simulink model "te_plant_network_controller"  (R2013b)
settings: Solver=ode5  SolverMode=SingleTasking  StartTime=0.0  StopTime=inf  FixedStep=Ts_base  MaxStep=Ts_base  MinStep=1e-6  RelTol=1e-6
InitFcn:
  | global model_type
  | model_type = 0
  | 
  | init_model
StopFcn:
  | %TEplot
values from neighbouring files (symbols this model uses):
  Dprocplc = 0    [init_model.m]
  Ts_actuator = repmat(Ts_scan,12,1)    [init_model.m]
  Ts_save = Ts_base    (= 0.000277777777778)    [init_model.m]
  Ts_scan = 30*Ts_base    (= 0.00833333333333)    [init_model.m]
  Ts_sensor = repmat(Ts_scan,41,1)    [init_model.m]
  xmeas_local_port_rx = xmeas_local_port_tx    [init_model.m]
  xmeas_local_port_tx = 9601:9699    [init_model.m]
  xmv_local_port_rx = xmv_local_port_tx    [init_model.m]
  xmv_local_port_tx = 9801:9899    [init_model.m]
libraries: TEsim_utils x8
settings Model: Creator=rnc4  LastModifiedBy=rnc4
settings DataIOCC: LimitDataPoints=off  LoadInitialState=on  SaveFinalState=on  SaveFormat=Structure  SignalLoggingSaveFormat=ModelDataLogs  SaveOutput=off  SaveTime=off  SignalLoggingName=sigsOut
settings OptimizationCC: InitFltsAndDblsToZero=on  SimCompilerOptimization=On
settings DebuggingCC: SaveWithParameterizedLinksMsg=none  SignalResolutionControl=TryResolveAllWithWarning  SolverPrmCheckMsg=none  MultiTaskDSMMsg=warning  MultiTaskCondExecSysMsg=none  FcnCallInpInsideContextMsg=UseLocalSettings
settings HardwareCC: TargetUnknown=on
settings RTWCC: IncludeERTFirstTime=on
settings GRTTargetCC: TargetFcnLib=ansi_tfl_tmw.mat  CodeReplacementLibrary=None  CombineOutputUpdateFcns=off  CPPClassGenCompliant=on  GRTInterface=on

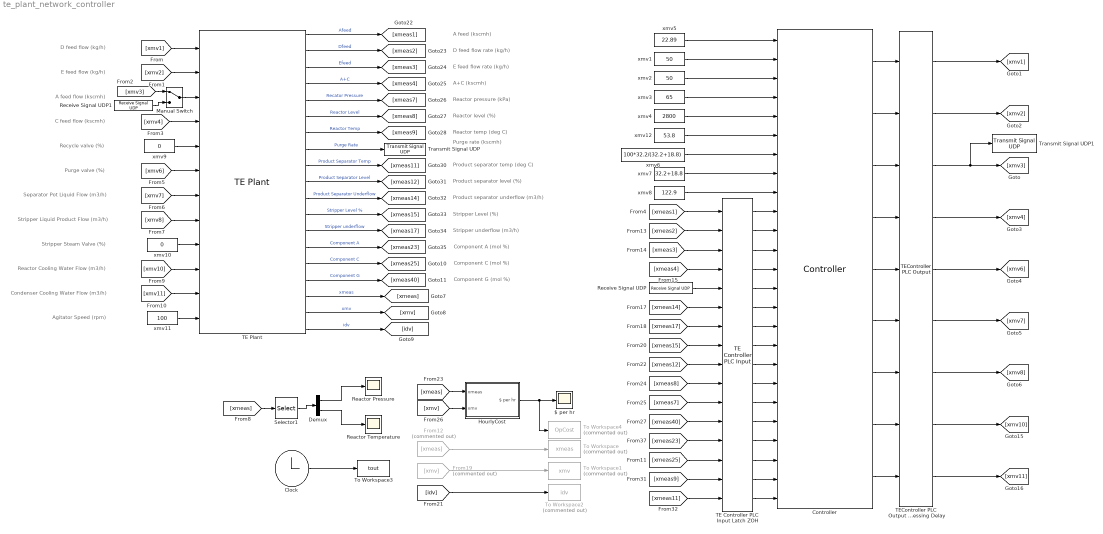
== system te_plant_network_controller ==
  note: Agitator Speed (rpm)
  note: Condenser Cooling Water Flow (m3/h)
  note: Reactor Cooling Water Flow (m3/h)
  note: Stripper Steam Valve (%)
  note: Stripper Liquid Product Flow (m3/h)
  note: Separator Pot Liquid Flow (m3/h)
  note: Purge valve (%)
  note: Recycle valve (%)
  note: C feed flow (kscmh)
  note: A feed flow (kscmh)
  note: E feed flow (kg/h)
  note: D feed flow (kg/h)
  note: Component G (mol %)
  note: Component C (mol %)
  note: Component A (mol %)
  note: Stripper underflow (m3/h)
  note: Stripper Level (%)
  note: Product separator underflow (m3/h)
  note: Product separator level (%)
  note: Product separator temp (deg C)
  note: Purge rate (kscmh)
  note: Reactor temp (deg C)
  note: Reactor level (%)
  note: Reactor pressure (kPa)
  note: A+C (kscmh)
  note: E feed flow rate (kg/h)
  note: D feed flow rate (kg/h)
  note: A feed (kscmh)
  $ per hr : Scope
      settings: YMin=75  YMax=400  SaveName=OpCost  SampleInput=on  SampleTime=Ts_save
  Clock : Clock
  Controller : TEsim_utils/TEsim/Controller
  Demux : Demux  Outputs=2
  From12 : From  Commented=on  GotoTag=xmeas
      settings: CloseFcn=tagdialog Close
  From19 : From  Commented=on  GotoTag=xmv
      settings: CloseFcn=tagdialog Close
  HourlyCost : Subsystem
  Manual Switch : ManualSwitch
  Reactor Pressure : Scope
      settings: TimeRange=30  YMin=0  YMax=3200  SampleInput=on  SampleTime=Ts_save
  Reactor Temperature : Scope
      settings: TimeRange=15  YMin=0  YMax=200  SampleInput=on  SampleTime=Ts_save
  Receive Signal UDP : TEsim_utils/Communications/Receive Signal UDP  Host=localhost  Port=remote_port  LocalPort=xmeas_local_port_rx(10)  SampleTime=Ts_sensor(10)
  Receive Signal UDP1 : TEsim_utils/Communications/Receive Signal UDP  Host=localhost  Port=remote_port  LocalPort=xmv_local_port_rx(3)  SampleTime=Ts_actuator(3)
  Selector1 : Selector  InputPortWidth=41  IndexOptions=Index vector (dialog)  Indices=[7 9]  OutputSizes=1
  TE Controller PLC Input Latch ZOH : TEsim_utils/PLC/TE Controller PLC Input  SampleTime=Ts_scan
  TE Plant : TEsim_utils/TEsim/TE Plant  SystemSampleTime=-1
  TEController PLC Output Processing Delay : TEsim_utils/PLC/TEController PLC Output  DelayTime=Dprocplc  InitialOutput=1
  To Workspace : ToWorkspace  Commented=on  VariableName=xmeas  SampleTime=Ts_save
  To Workspace1 : ToWorkspace  Commented=on  VariableName=xmv  SampleTime=Ts_save
  To Workspace2 : ToWorkspace  Commented=on  VariableName=idv  SampleTime=Ts_save
  To Workspace3 : ToWorkspace  VariableName=tout  SampleTime=Ts_save
  To Workspace4 : ToWorkspace  Commented=on  VariableName=OpCost  SampleTime=Ts_save
  Transmit Signal UDP : TEsim_utils/Communications/Transmit Signal UDP  Ts=Ts_sensor(10)  Host=localhost  Port=remote_port  LocalPort=xmeas_local_port_tx(10)  EnableBlockingMode=on
  Transmit Signal UDP1 : TEsim_utils/Communications/Transmit Signal UDP  Ts=Ts_actuator(3)  Host=localhost  Port=remote_port  LocalPort=xmv_local_port_tx(3)  EnableBlockingMode=on
  xmv1 : Constant  Value=50
  xmv10 : Constant  Value=0
  xmv11 : Constant  Value=100
  xmv12 : Constant  Value=53.8
  xmv2 : Constant  Value=50
  xmv3 : Constant  Value=65
  xmv4 : Constant  Value=2800
  xmv5 : Constant  Value=22.89
  xmv6 : Constant  Value=100*32.2/(32.2+18.8)
  xmv7 : Constant  Value=32.2+18.8
  xmv8 : Constant  Value=122.9
  xmv9 : Constant  Value=0
  wires:
  Clock/1 -> To Workspace3/1
  HourlyCost/1($ per hr) -> To Workspace4/1, $ per hr/1
  xmv8/1 -> Controller/9
  xmv7/1 -> Controller/8
  xmv6/1 -> Controller/7
  xmv12/1 -> Controller/6
  xmv4/1 -> Controller/5
  xmv3/1 -> Controller/4
  xmv2/1 -> Controller/3
  xmv1/1 -> Controller/2
  xmv5/1 -> Controller/1
  TE Plant/7 -> [xmeas9]  "Reactor Temp"
  TE Plant/5 -> [xmeas7]  "Recator Pressure"
  TE Plant/18 -> [xmv]  "xmv"
  TE Plant/17 -> [xmeas]  "xmeas"
  [xmv1] -> TE Plant/1
  [xmv2] -> TE Plant/2
  [xmv4] -> TE Plant/4
  xmv9/1 -> TE Plant/5
  [xmv6] -> TE Plant/6
  [xmv7] -> TE Plant/7
  [xmv8] -> TE Plant/8
  xmv10/1 -> TE Plant/9
  [xmv10] -> TE Plant/10
  [xmv11] -> TE Plant/11
  xmv11/1 -> TE Plant/12
  TE Plant/2 -> [xmeas2]  "Dfeed"
  TE Plant/3 -> [xmeas3]  "Efeed"
  TE Plant/4 -> [xmeas4]  "A+C"
  TE Plant/6 -> [xmeas8]  "Reactor Level"
  TE Plant/8 -> Transmit Signal UDP/1  "Purge Rate"
  TE Plant/9 -> [xmeas11]  "Product Separator Temp"
  TE Plant/10 -> [xmeas12]  "Product Separator Level"
  TE Plant/11 -> [xmeas14]  "Product Separator Underflow"
  TE Plant/12 -> [xmeas15]  "Stripper Level %"
  TE Plant/13 -> [xmeas17]  "Stripper underflow"
  TE Plant/14 -> [xmeas23]  "Component A"
  TE Plant/15 -> [xmeas25]  "Component C"
  TE Plant/16 -> [xmeas40]  "Component G"
  TE Plant/19 -> [idv]  "idv"
  From12/1 -> To Workspace/1
  From19/1 -> To Workspace1/1
  [idv] -> To Workspace2/1
  [xmeas] -> HourlyCost/1(xmeas)
  [xmv] -> HourlyCost/2(xmv)
  TE Plant/1 -> [xmeas1]  "Afeed"
  [xmeas] -> Selector1/1
  Selector1/1 -> Demux/1
  Demux/1 -> Reactor Pressure/1
  Demux/2 -> Reactor Temperature/1
  Manual Switch/1 -> TE Plant/3
  [xmv3] -> Manual Switch/1
  Receive Signal UDP1/1 -> Manual Switch/2
  TE Controller PLC Input Latch ZOH/7 -> Controller/16
  TE Controller PLC Input Latch ZOH/6 -> Controller/15
  TE Controller PLC Input Latch ZOH/12 -> Controller/21
  TE Controller PLC Input Latch ZOH/2 -> Controller/11
  TE Controller PLC Input Latch ZOH/13 -> Controller/22
  TE Controller PLC Input Latch ZOH/5 -> Controller/14
  TE Controller PLC Input Latch ZOH/8 -> Controller/17
  TE Controller PLC Input Latch ZOH/10 -> Controller/19
  TE Controller PLC Input Latch ZOH/16 -> Controller/25
  TE Controller PLC Input Latch ZOH/14 -> Controller/23
  TE Controller PLC Input Latch ZOH/9 -> Controller/18
  TE Controller PLC Input Latch ZOH/1 -> Controller/10
  TE Controller PLC Input Latch ZOH/4 -> Controller/13
  TE Controller PLC Input Latch ZOH/11 -> Controller/20
  TE Controller PLC Input Latch ZOH/3 -> Controller/12
  TE Controller PLC Input Latch ZOH/15 -> Controller/24
  Receive Signal UDP/1 -> TE Controller PLC Input Latch ZOH/5
  [xmeas17] -> TE Controller PLC Input Latch ZOH/7
  [xmeas14] -> TE Controller PLC Input Latch ZOH/6
  [xmeas4] -> TE Controller PLC Input Latch ZOH/4
  [xmeas8] -> TE Controller PLC Input Latch ZOH/10
  [xmeas12] -> TE Controller PLC Input Latch ZOH/9
  [xmeas15] -> TE Controller PLC Input Latch ZOH/8
  [xmeas25] -> TE Controller PLC Input Latch ZOH/14
  [xmeas7] -> TE Controller PLC Input Latch ZOH/11
  [xmeas23] -> TE Controller PLC Input Latch ZOH/13
  [xmeas11] -> TE Controller PLC Input Latch ZOH/16
  [xmeas9] -> TE Controller PLC Input Latch ZOH/15
  [xmeas40] -> TE Controller PLC Input Latch ZOH/12
  [xmeas3] -> TE Controller PLC Input Latch ZOH/3
  [xmeas2] -> TE Controller PLC Input Latch ZOH/2
  [xmeas1] -> TE Controller PLC Input Latch ZOH/1
  Controller/1 -> TEController PLC Output Processing Delay/1
  Controller/2 -> TEController PLC Output Processing Delay/2
  Controller/3 -> TEController PLC Output Processing Delay/3
  Controller/4 -> TEController PLC Output Processing Delay/4
  Controller/5 -> TEController PLC Output Processing Delay/5
  Controller/6 -> TEController PLC Output Processing Delay/6
  Controller/7 -> TEController PLC Output Processing Delay/7
  Controller/8 -> TEController PLC Output Processing Delay/8
  Controller/9 -> TEController PLC Output Processing Delay/9
  TEController PLC Output Processing Delay/1 -> [xmv1]
  TEController PLC Output Processing Delay/2 -> [xmv2]
  TEController PLC Output Processing Delay/3 -> Transmit Signal UDP1/1, [xmv3]
  TEController PLC Output Processing Delay/4 -> [xmv4]
  TEController PLC Output Processing Delay/5 -> [xmv6]
  TEController PLC Output Processing Delay/6 -> [xmv7]
  TEController PLC Output Processing Delay/7 -> [xmv8]
  TEController PLC Output Processing Delay/8 -> [xmv10]
  TEController PLC Output Processing Delay/9 -> [xmv11]

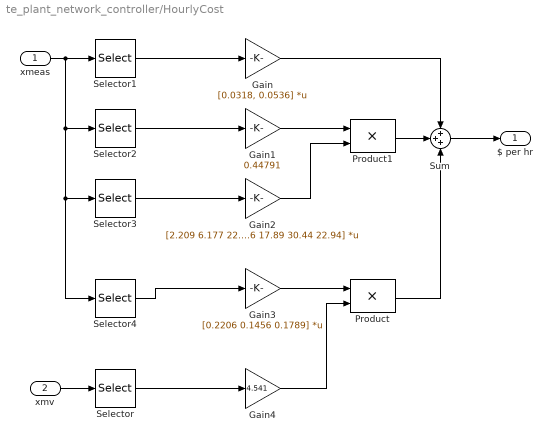
== system te_plant_network_controller/HourlyCost ==
  xmeas : Inport  PortDimensions=41
  xmv : Inport  Port=2  PortDimensions=12
  Gain : Gain  Gain=[0.0318, 0.0536]  Multiplication=Matrix(K*u)  SaturateOnIntegerOverflow=on  OutDataTypeStr=Inherit: Same as input  ParamDataTypeStr=Inherit: Same as input
      settings: AttributesFormatString=%<Gain>
  Gain1 : Gain  Gain=0.44791  SaturateOnIntegerOverflow=on  OutDataTypeStr=Inherit: Same as input  ParamDataTypeStr=Inherit: Same as input
      settings: AttributesFormatString=%<Gain>
  Gain2 : Gain  Gain=[2.209 6.177 22.06 14.56 17.89 30.44 22.94]  Multiplication=Matrix(K*u)  SaturateOnIntegerOverflow=on  OutDataTypeStr=Inherit: Same as input  ParamDataTypeStr=Inherit: Same as input
      settings: AttributesFormatString=%<Gain>
  Gain3 : Gain  Gain=[0.2206 0.1456 0.1789]  Multiplication=Matrix(K*u)  SaturateOnIntegerOverflow=on  OutDataTypeStr=Inherit: Same as input  ParamDataTypeStr=Inherit: Same as input
      settings: AttributesFormatString=%<Gain>
  Gain4 : Gain  Gain=4.541  SaturateOnIntegerOverflow=on  OutDataTypeStr=Inherit: Same as input  ParamDataTypeStr=Inherit: Same as input
      settings: AttributesFormatString=%<Gain>
  Product : Product  SaturateOnIntegerOverflow=on  OutDataTypeStr=Inherit: Same as first input
  Product1 : Product  SaturateOnIntegerOverflow=on  OutDataTypeStr=Inherit: Same as first input
  Selector : Selector  InputPortWidth=12  IndexOptions=Index vector (dialog)  Indices=8  OutputSizes=1
  Selector1 : Selector  InputPortWidth=41  IndexOptions=Index vector (dialog)  Indices=[19 20]  OutputSizes=1
  Selector2 : Selector  InputPortWidth=41  IndexOptions=Index vector (dialog)  Indices=[10]  OutputSizes=1
  Selector3 : Selector  InputPortWidth=41  IndexOptions=Index vector (dialog)  Indices=[29, 31:36]  OutputSizes=1
  Selector4 : Selector  InputPortWidth=41  IndexOptions=Index vector (dialog)  Indices=[37:39]  OutputSizes=1
  Sum : Sum  Inputs=+++  SaturateOnIntegerOverflow=on
  $ per hr : Outport
  wires:
  xmv/1 -> Selector/1
  xmeas/1 -> Selector1/1, Selector2/1, Selector3/1, Selector4/1
  Selector1/1 -> Gain/1
  Selector2/1 -> Gain1/1
  Selector3/1 -> Gain2/1
  Selector4/1 -> Gain3/1
  Selector/1 -> Gain4/1
  Gain3/1 -> Product/1
  Gain4/1 -> Product/2
  Sum/1 -> $ per hr/1
  Product/1 -> Sum/3
  Gain/1 -> Sum/1
  Product1/1 -> Sum/2
  Gain1/1 -> Product1/1
  Gain2/1 -> Product1/2
